simulink library "calculatePathSpeed_ul"  (R2018b)
settings: Solver=VariableStepAuto  StartTime=0.0  StopTime=10.0  RelTol=1e-3
undefined symbols (not defined in the file or in its folder): pathHeight_m, pathWidth_m
settings Model: Creator=mcobb  LastModifiedBy=mcobb
settings DebuggingCC: LibraryContextMissingDiagnostic=none
settings SFSimCC: SimUseLocalCustomCode=off
settings RTWCC: RTWUseLocalCustomCode=off

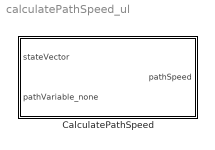
== system calculatePathSpeed_ul ==
  CalculatePathSpeed : Subsystem

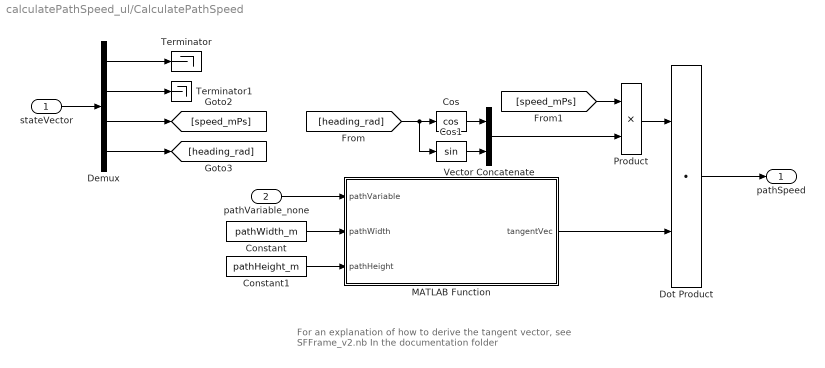
== system calculatePathSpeed_ul/CalculatePathSpeed ==
  note: For an explanation of how to derive the tangent vector, see
      | SFFrame_v2.nb
      | In the documentation folder
  stateVector : Inport
  pathVariable_none : Inport  Port=2
  Constant : Constant  Value=pathWidth_m
  Constant1 : Constant  Value=pathHeight_m
  Cos : Trigonometry  Operator=cos
  Cos1 : Trigonometry
  Demux : Demux
  Dot Product : DotProduct  InputSameDT=on  OutDataTypeStr=Inherit: Inherit via internal rule
  MATLAB Function : MATLAB Function  TreatAsAtomicUnit=on
  Product : Product
  Terminator : Terminator
  Terminator1 : Terminator
  Vector Concatenate : Concatenate
  pathSpeed : Outport  PortDimensions=1
  wires:
  stateVector/1 -> Demux/1
  Demux/1 -> Terminator/1
  Demux/2 -> Terminator1/1
  Demux/3 -> [speed_mPs]
  Demux/4 -> [heading_rad]
  [heading_rad] -> Cos/1, Cos1/1
  Cos/1 -> Vector Concatenate/1
  Cos1/1 -> Vector Concatenate/2
  Vector Concatenate/1 -> Product/2
  [speed_mPs] -> Product/1
  Product/1 -> Dot Product/1
  pathVariable_none/1 -> MATLAB Function/1(pathVariable)
  Constant/1 -> MATLAB Function/2(pathWidth)
  Constant1/1 -> MATLAB Function/3(pathHeight)
  MATLAB Function/1(tangentVec) -> Dot Product/2
  Dot Product/1 -> pathSpeed/1

== matlab function calculatePathSpeed_ul/CalculatePathSpeed/MATLAB Function ==
  data: pathVariable input; tangentVec output size=[1 2]; pathWidth input; pathHeight input
function tangentVec = fcn(pathVariable,pathWidth,pathHeight)
coder.extrinsic('calculatePathTangentVector');
tangentVec = [NaN NaN];
tangentVec = calculatePathTangentVector(pathVariable,pathWidth,pathHeight);
end
